simulink model "MinMax"  (R2017b)
settings: Solver=FixedStepDiscrete  StartTime=0.0  StopTime=10.0  FixedStep=0.200000  RelTol=1e-3  EnableMultiTasking=on
model workspace (MAT data in the model file):
  input_struct.time = [0; 0.2; 0.4; 0.6; 0.8; 1; 1.2; 1.4; 1.6; 1.8; 2; 2.2; 2.4; 2.6; 2.8; 3; 3.2; 3.4; 3.6; 3.8; 4; 4.2; 4.4; 4.6; 4.8; 5; 5.2; 5.4; 5.6; 5.8; 6; 6.2; 6.4; 6.6; 6.8; 7; 7.2; 7.4; 7.6; 7.8; 8; 8.2; 8.4; 8.6; 8.8; 9; 9.2; 9.4; 9.6; 9.8; 10; 10.2; 10.4; 10.6; 10.8; 11; 11.2; 11.4; 11.6; 11.8; 12; 12.2; 12.4; 12.6; 12.8; 13; 13.2; 13.4; 13.6; 13.8; 14; 14.2; 14.4; 14.6; 14.8; 15; 15.2; 15.4; 15.6; 15.8; 16; 16.2; 16.4; 16.6; 16.8; 17; 17.2; 17.4; 17.6; 17.8; 18; 18.2; 18.4; 18.6; 18.8; 19; 19.2; 19.4; 19.6; 19.8]
  input_struct.signals.name = 'In1'
  input_struct.signals.values = [81.6576449529; 90.6734017705; 13.5716948131; 91.4242097578; 63.6035653763; 10.6565000949; 28.5713236678; 55.1412704013; 95.793176708; 96.5239649847; 16.6036950861; 97.0886853943; 95.7595278761; 49.0521892236; 80.22776642; 15.0467475241; 42.75436698; 91.6578169937; 79.4285256264; 95.9897502129; 65.9183292165; 4.53545617884; 85.063801281; 93.465331528; 68.1947803309; 76.0162729273; 74.5701143444; 39.8304749339; 65.8923111276; 17.9474820933; 70.8985627139; 4.15145179136; 28.4153755111; 5.57096767248; 10.6160463423; 82.5223250044; 69.7880336746; 32.392848526; 95.071982835; 4.41016196979; 44.435691606; 38.7742872522; 76.7861620268; 79.7247902126; 19.5003878509; 49.486675183; 45.1130338704; 64.984988001; 71.2271182549; 75.7139815163; 28.3264826229; 68.2905650085; 65.8547023934; 17.0985617843; 12.7807704743; 50.3380411462; 96.0146518931; 34.6981869399; 58.941507347; 23.1573820096; 75.3754388713; 26.2544164305; 51.0897481148; 70.208595543; 89.199422001; 95.9698510953; 55.1743374664; 14.72381984; 15.7801065503; 26.4933171582; 84.2310083424; 26.1739357182; 81.6141977808; 25.1089719038; 92.9970986955; 35.6483928325; 20.4629297927; 25.8573019396; 61.9884229385; 47.8555960414; 35.8142911992; 83.2520341617; 58.9411450241; 55.4226372208; 91.8021727192; 29.2980628632; 75.962822682; 75.6191803336; 38.6641388506; 57.2143424318; 8.50957466674; 6.34106174799; 53.5489577479; 78.1375557801; 93.4670577387; 13.8607146389; 57.3135424263; 47.4696734648; 2.17830488062; 34.3751417955]
  input_struct.signals.dimensions = 1
settings Model: Creator=hbourbou  LastModifiedBy=hbourbou
settings DataIOCC: LimitDataPoints=on  SaveFormat=Structure
settings OptimizationCC: LifeSpan=inf
settings DebuggingCC: SFUnexpectedBacktrackingDiag=warning  SFNoUnconditionalDefaultTransitionDiag=warning  SFExecutionAtInitializationDiag=none
settings HardwareCC: ProdBitPerPointer=32  ProdBitPerSizeT=32  ProdBitPerPtrDiffT=32  ProdLargestAtomicFloat=None  ProdIntDivRoundTo=Undefined  ProdEndianess=Unspecified  ProdWordSize=32  ProdHWDeviceType=32-bit Generic
settings ModelReferenceCC: PropagateSignalLabelsOutOfModel=off
settings CodeAppCC: StateflowObjectComments=on
settings GRTTargetCC: TargetLangStandard=C89/C90 (ANSI)  GeneratePreprocessorConditionals=Disable all
settings ConfigComp: CovMetricSettings=dw  CovHtmlReporting=on  CovSaveCumulativeToWorkspaceVar=on  CovSaveSingleToWorkspaceVar=on  CovExternalEMLEnable=off

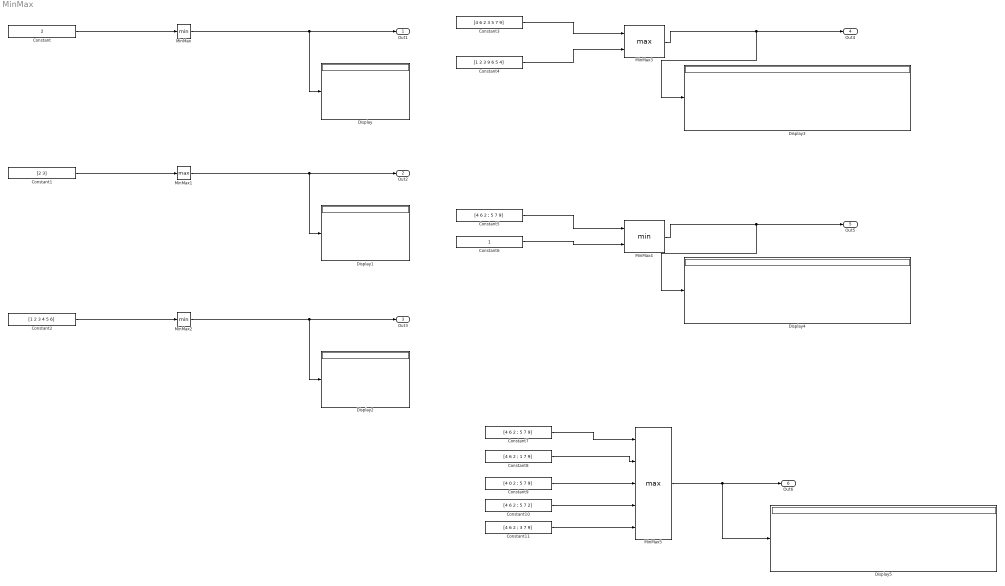
== system MinMax ==
  Constant : Constant  Value=2
  Constant1 : Constant  Value=[2 3]  OutDataTypeStr=int32
  Constant10 : Constant  Value=[4 6 2 ; 5 7 2]
  Constant11 : Constant  Value=[4 6 2 ; 3 7 9]
  Constant2 : Constant  Value=[1 2 3 4 5 6]
  Constant3 : Constant  Value=[4 6 2 3 5 7 9]
  Constant4 : Constant  Value=[1 2 3 9 6 5 4]
  Constant5 : Constant  Value=[4 6 2 ; 5 7 9]
  Constant6 : Constant
  Constant7 : Constant  Value=[4 6 2 ; 5 7 9]
  Constant8 : Constant  Value=[4 6 2 ; 1 7 9]
  Constant9 : Constant  Value=[4 0 2 ; 5 7 9]
  Display{,1..5} (6 alike) : Display
  MinMax : MinMax
  MinMax1 : MinMax  Function=max
  MinMax2 : MinMax
  MinMax3 : MinMax  Function=max  Inputs=2
  MinMax4 : MinMax  Inputs=2
  MinMax5 : MinMax  Function=max  Inputs=5
  Out1 : Outport
  Out2 : Outport  Port=2
  Out3 : Outport  Port=3
  Out4 : Outport  Port=4
  Out5 : Outport  Port=5
  Out6 : Outport  Port=6
  wires:
  Constant/1 -> MinMax/1
  MinMax/1 -> Display/1, Out1/1
  Constant1/1 -> MinMax1/1
  MinMax1/1 -> Display1/1, Out2/1
  Constant2/1 -> MinMax2/1
  MinMax2/1 -> Display2/1, Out3/1
  Constant3/1 -> MinMax3/1
  MinMax3/1 -> Display3/1, Out4/1
  Constant4/1 -> MinMax3/2
  Constant5/1 -> MinMax4/1
  MinMax4/1 -> Display4/1, Out5/1
  Constant6/1 -> MinMax4/2
  Constant7/1 -> MinMax5/1
  Constant8/1 -> MinMax5/2
  Constant9/1 -> MinMax5/3
  Constant10/1 -> MinMax5/4
  Constant11/1 -> MinMax5/5
  MinMax5/1 -> Display5/1, Out6/1
